simulink model "Power_electronics_ProjB"  (R2024b)
settings: Solver=VariableStepAuto  StartTime=0.0  StopTime=0.1  RelTol=1e-3
libraries: spsACCurrentSourceLib x3, spsFourierLib x2, spsParallelRLCBranchLib x2, spsCurrentMeasurementLib x1, spsGroundLib x1, spsVoltageMeasurementLib x1, sps_lib x1
settings Model: Creator=MTMTAD006  LastModifiedBy=MTMTAD006

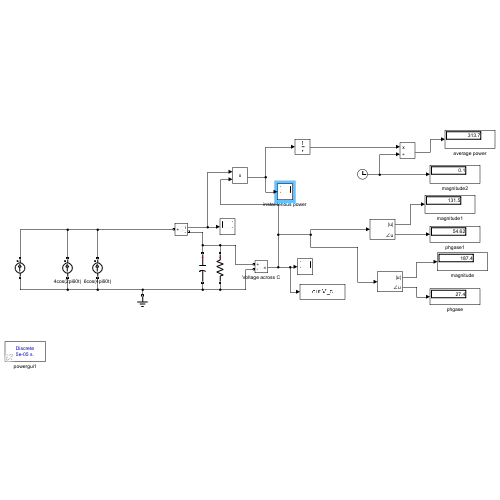
[thumbnail: Simulink's stored preview of the top-level diagram]
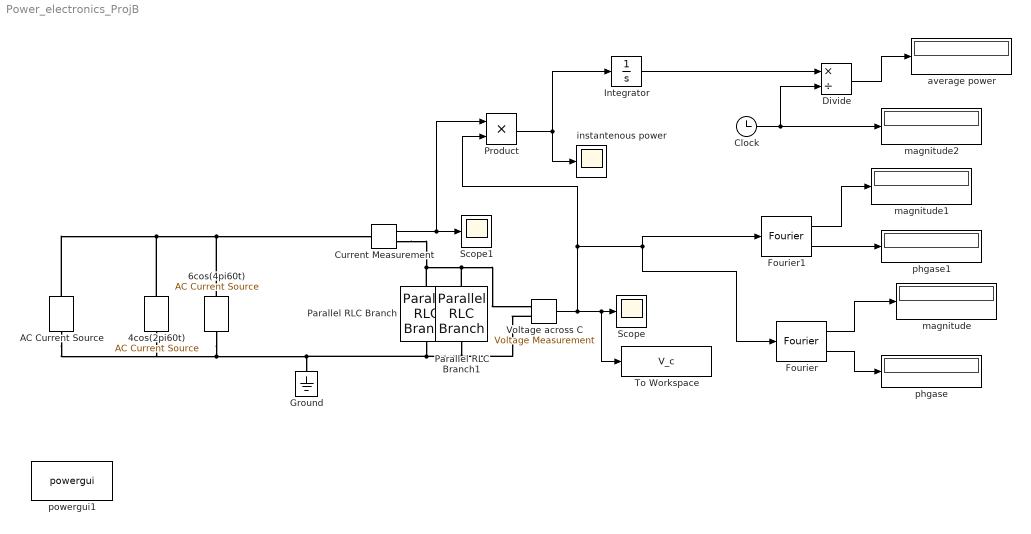
== system Power_electronics_ProjB ==
  4cos(2pi60t) : spsACCurrentSourceLib/AC Current Source  Amplitude=4  Phase=90  Frequency=60  SampleTime=0  Measurements=None
      settings: LibrarySourceBlock=sps_lib/Sources/AC Current Source
  6cos(4pi60t) : spsACCurrentSourceLib/AC Current Source  Amplitude=6  Phase=90  Frequency=120  SampleTime=0  Measurements=None
      settings: LibrarySourceBlock=sps_lib/Sources/AC Current Source
  AC Current Source : spsACCurrentSourceLib/AC Current Source  Amplitude=3  Phase=0  Frequency=0  SampleTime=0  Measurements=None
      settings: LibrarySourceBlock=sps_lib/Sources/AC Current Source
  Clock : Clock
  Current Measurement : spsCurrentMeasurementLib/Current Measurement  PhasorSimulation=off  OutputType=Complex  PSBequivalent=0
  Divide : Product  Inputs=*/
  Fourier : spsFourierLib/Fourier  Freq=60  n=1  InInit=[0, 0]  Ts=0
  Fourier1 : spsFourierLib/Fourier  Freq=120  n=1  InInit=[0, 0]  Ts=0
  Ground : spsGroundLib/Ground  LConnTagsString=a
  Integrator : Integrator
  Parallel RLC Branch : spsParallelRLCBranchLib/Parallel RLC Branch  LConnTagsString=a  RConnTagsString=__new0  BranchType=C  Resistance=100  Inductance=1e-3  SetiL0=off  InitialCurrent=0  Capacitance=50e-6  Setx0=off  InitialVoltage=0  Measurements=None
  Parallel RLC Branch1 : spsParallelRLCBranchLib/Parallel RLC Branch  LConnTagsString=a  RConnTagsString=__new0  BranchType=R  Resistance=100  Inductance=1e-3  SetiL0=off  InitialCurrent=0  Capacitance=50e-6  Setx0=off  InitialVoltage=0  Measurements=None
  Product : Product
  Scope : Scope
  Scope1 : Scope
  To Workspace : ToWorkspace  VariableName=V_c  SaveFormat=Structure With Time  SampleTime=-1
  Voltage across C : spsVoltageMeasurementLib/Voltage Measurement  PhasorSimulation=off  OutputType=Complex  PSBequivalent=0
  average power : Display
      settings: Decimation=2
  instantenous power : Scope
  magnitude : Display
      settings: Decimation=2
  magnitude1 : Display
      settings: Decimation=2
  magnitude2 : Display
      settings: Decimation=2
  phgase : Display
      settings: Decimation=2
  phgase1 : Display
      settings: Decimation=2
  powergui1 : sps_lib/powergui  Priority=1  SimulationMode=Discrete  SampleTime=50e-6  frequency=60  Iterations=50  frequencyindice=0  Pbase=100e6  ErrMax=1e-4  UnitsV=kV  UnitsW=MW  buscounter=0  FunctionMessages=off  echomessages=off  EnableUseOfTLC=off  CurrentSourceSwitches=off  DisableSnubberDevices=off  DisableRonSwitches=off  DisableVfSwitches=off  DisplayEquations=off  AutomaticDiscreteSolvers=off  SolverType=Tustin/Backward Euler (TBE)  Interpol=off  ExternalGateDelay=off  methode=off  Ts=100  x0status=blocks  SPID=on  SwTol=0  HookPort=off  NonlinearTolerance=1e-4  nMaxIteration=100  ContinueOnMaxIteration=off  RestoreLinks=warning  ResistiveCurrentMeasurement=off  Frange=[0:2:500]  Ylog=off  Xlog=on  ShowGrid=off  save=off  variable=ZData  structure=0  ZoomFFT=off  StartTime=0.0  cycles=1  DisplayStyle=1  fundamental=60  FreqAxis=off  MaxFrequency=1000  frequencyindicesteady=1  RmsSteady=1  display=off
  wires:
  Voltage across C/1 -> Product/2, Fourier/1, Fourier1/1, To Workspace/1, Scope/1
  Current Measurement/1 -> Product/1, Scope1/1
  Fourier/1 -> magnitude/1
  Fourier/2 -> phgase/1
  Fourier1/1 -> magnitude1/1
  Fourier1/2 -> phgase1/1
  Product/1 -> Integrator/1, instantenous power/1
  Clock/1 -> magnitude2/1, Divide/2
  Integrator/1 -> Divide/1
  Divide/1 -> average power/1
  connections:
  Voltage across C/LConn2 -- Parallel RLC Branch1/RConn1 -- Parallel RLC Branch/RConn1 -- 6cos(4pi60t)/LConn1 -- 4cos(2pi60t)/LConn1 -- AC Current Source/LConn1 -- Ground/LConn1
  AC Current Source/RConn1 -- 4cos(2pi60t)/RConn1 -- 6cos(4pi60t)/RConn1 -- Current Measurement/LConn1
  Current Measurement/RConn1 -- Parallel RLC Branch/LConn1 -- Parallel RLC Branch1/LConn1 -- Voltage across C/LConn1
